simulink model "robot_arm_simul_utilization"  (R2017a)
settings: Solver=ode4  StartTime=0.0  StopTime=simul_time  FixedStep=delta  RelTol=1e-3
values from neighbouring files (symbols this model uses):
  B = 0    [Plot_utilization.m]
undefined symbols (not defined in the file or in its folder): A, A_, B_, C, C_, D, D_, delta, Dis_instant_P1, Dis_instant_P2, Dis_interval_P1, Dis_interval_P2, Dis_size_P1, Dis_size_P2, K, K_, L, L_, ref_P1, ref_P2
settings Model: Creator=sihoon  LastModifiedBy=root

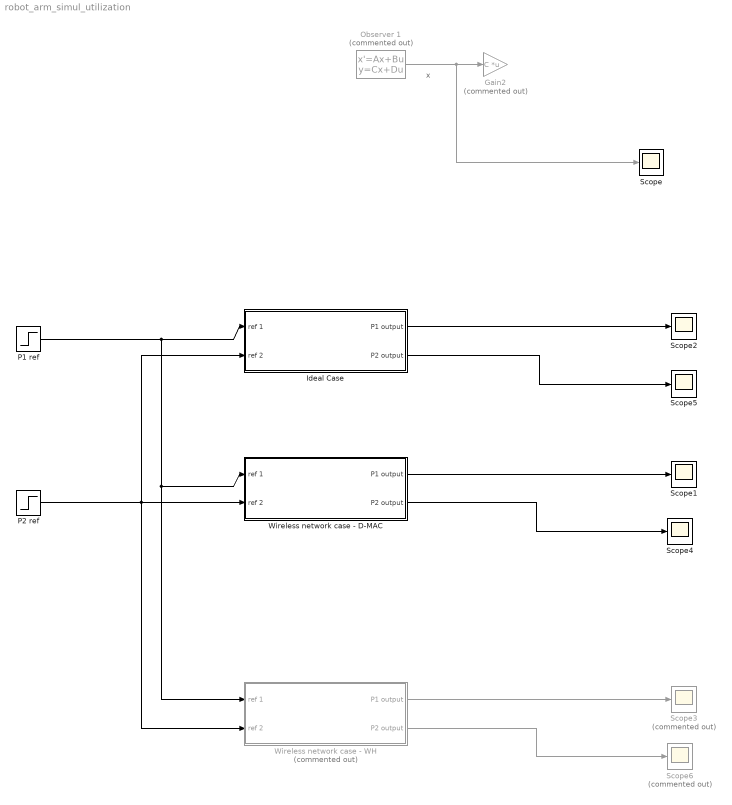
== system robot_arm_simul_utilization ==
  note: x
  Gain2 : Gain  Commented=on  Gain=C  Multiplication=Matrix(K*u)
  Ideal Case : Subsystem
  Observer 1 : StateSpace  Commented=on  A=A  B=B  C=eye(2)  D=[0; 0]  X0=0
  P1 ref : Step  Time=0  After=ref_P1  SampleTime=0
  P2 ref : Step  Time=0  After=ref_P2  SampleTime=0
  Scope{,1..2,4..5} (5 alike) : Scope
  Scope3 : Scope  Commented=on
  Scope6 : Scope  Commented=on
  Wireless network case - D-MAC : Subsystem
  "Wireless network case - WH " : Subsystem  Commented=on
  wires:
  Observer 1/1 -> Scope/1, Gain2/1
  Ideal Case/1(P1 output) -> Scope2/1
  Wireless network case - D-MAC/1(P1 output) -> Scope1/1
  P1 ref/1 -> "Wireless network case - WH "/1(ref 1), Wireless network case - D-MAC/1(ref 1), Ideal Case/1(ref 1)
  Wireless network case - D-MAC/2(P2 output) -> Scope4/1
  P2 ref/1 -> "Wireless network case - WH "/2(ref 2), Ideal Case/2(ref 2), Wireless network case - D-MAC/2(ref 2)
  Ideal Case/2(P2 output) -> Scope5/1
  "Wireless network case - WH "/1(P1 output) -> Scope3/1
  "Wireless network case - WH "/2(P2 output) -> Scope6/1

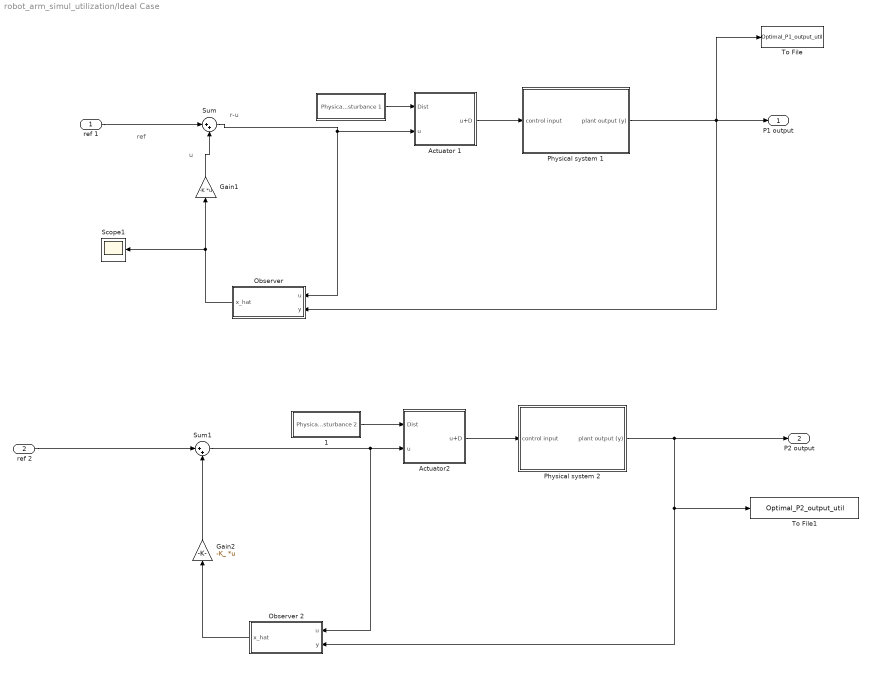
== system robot_arm_simul_utilization/Ideal Case ==
  note: u
  note: ref
  note: r-u
  ref 1 : Inport
  ref 2 : Inport  Port=2
  " " : Subsystem
  " 1" : Subsystem
  Actuator 1 : Subsystem
  Actuator2 : Subsystem
  Gain1 : Gain  Gain=-K  Multiplication=Matrix(K*u)
  Gain2 : Gain  Gain=-K_  Multiplication=Matrix(K*u)
  Observer : Subsystem
  Observer 2 : Subsystem
  Physical system 1 : Subsystem
  Physical system 2 : Subsystem
  Scope1 : Scope
  Sum : Sum  Inputs=|++
  Sum1 : Sum  Inputs=|++
  To File : ToFile  Filename=Optimal_P1_output_util  SaveFormat=Timeseries
  To File1 : ToFile  Filename=Optimal_P2_output_util  SaveFormat=Timeseries
  P1 output : Outport
  P2 output : Outport  Port=2
  wires:
  Physical system 1/1(plant output (y)) -> Observer/2(y), To File/1, P1 output/1
  Observer/1(x_hat) -> Scope1/1, Gain1/1
  ref 1/1 -> Sum/1
  Gain1/1 -> Sum/2
  Sum/1 -> Actuator 1/2(u), Observer/1(u)
  Actuator 1/1(u+D) -> Physical system 1/1(control input)
  " "/1(Physical Disturbance 1) -> Actuator 1/1(Dist)
  Actuator2/1(u+D) -> Physical system 2/1(control input)
  " 1"/1(Physical Disturbance 2) -> Actuator2/1(Dist)
  Physical system 2/1(plant output (y)) -> Observer 2/2(y), To File1/1, P2 output/1
  ref 2/1 -> Sum1/1
  Gain2/1 -> Sum1/2
  Observer 2/1(x_hat) -> Gain2/1
  Sum1/1 -> Observer 2/1(u), Actuator2/2(u)

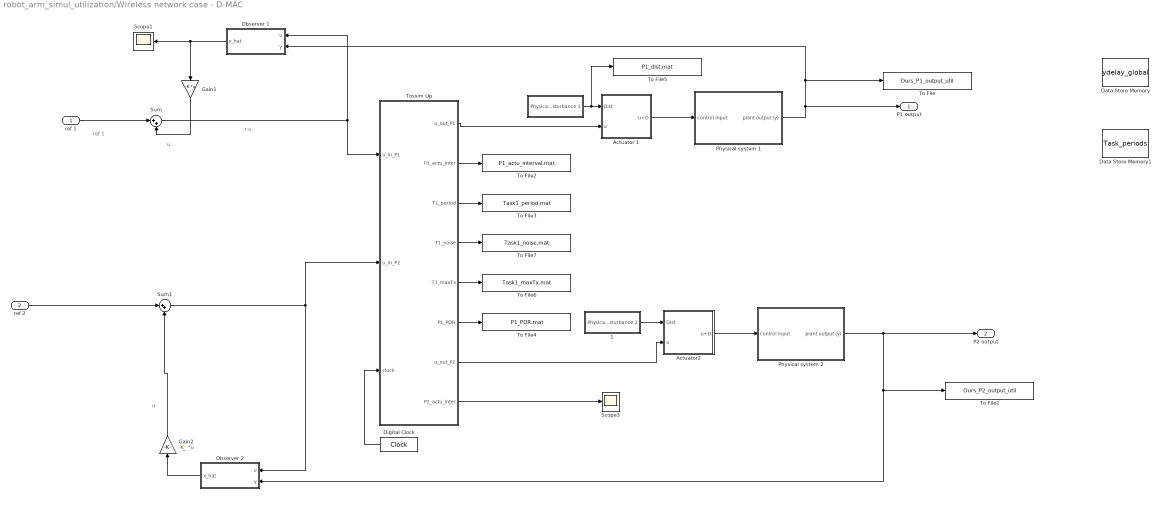
== system robot_arm_simul_utilization/Wireless network case - D-MAC ==
  note: u
  note: ref 1
  note: r-u
  note: u
  ref 1 : Inport
  ref 2 : Inport  Port=2
  " " : Subsystem
  " 1" : Subsystem
  Actuator 1 : Subsystem
  Actuator2 : Subsystem
  Data Store Memory : DataStoreMemory  DataStoreName=ydelay_global  ReadBeforeWriteMsg=warning  WriteAfterWriteMsg=warning  WriteAfterReadMsg=warning  InitialValue=[1; 1; 1; 1; 1; 1; 1; 1; 1; 1; 1; 1; 1; 1; 1]  ShowAdditionalParam=off  OutDataTypeStr=uint32
  Data Store Memory1 : DataStoreMemory  DataStoreName=Task_periods  ReadBeforeWriteMsg=warning  WriteAfterWriteMsg=warning  WriteAfterReadMsg=warning  InitialValue=Task_periods  ShowAdditionalParam=off  OutDataTypeStr=double
  Digital Clock : DigitalClock  SampleTime=delta
  Gain1 : Gain  Gain=-K  Multiplication=Matrix(K*u)
  Gain2 : Gain  Gain=-K_  Multiplication=Matrix(K*u)
  Observer 1 : Subsystem
  Observer 2 : Subsystem
  Physical system 1 : Subsystem
  Physical system 2 : Subsystem
  Scope1 : Scope
  Scope3 : Scope
  Sum : Sum  Inputs=|++
  Sum1 : Sum  Inputs=|++
  To File : ToFile  Filename=Ours_P1_output_util  SaveFormat=Timeseries
  To File1 : ToFile  Filename=Ours_P2_output_util  SaveFormat=Timeseries
  To File2 : ToFile  Filename=P1_actu_interval.mat  SaveFormat=Timeseries
  To File3 : ToFile  Filename=Task1_period.mat  SaveFormat=Timeseries
  To File4 : ToFile  Filename=P1_PDR.mat  SaveFormat=Timeseries
  To File5 : ToFile  Filename=P1_dist.mat  SaveFormat=Timeseries
  To File6 : ToFile  Filename=Task1_maxTx.mat  SaveFormat=Timeseries
  To File7 : ToFile  Filename=Task1_noise.mat  SaveFormat=Timeseries
  Tossim Up : MATLAB Function  TreatAsAtomicUnit=on
  P1 output : Outport
  P2 output : Outport  Port=2
  wires:
  ref 1/1 -> Sum/1
  Sum/1 -> Observer 1/1(u), Tossim Up/1(u_in_P1)
  Physical system 1/1(plant output (y)) -> Observer 1/2(y), To File/1, P1 output/1
  Gain1/1 -> Sum/2
  Observer 1/1(x_hat) -> Scope1/1, Gain1/1
  Tossim Up/7(u_out_P2) -> Actuator2/2(u)
  Digital Clock/1 -> Tossim Up/3(clock)
  Tossim Up/1(u_out_P1) -> Actuator 1/2(u)
  Actuator 1/1(u+D) -> Physical system 1/1(control input)
  " "/1(Physical Disturbance 1) -> To File5/1, Actuator 1/1(Dist)
  " 1"/1(Physical Disturbance 2) -> Actuator2/1(Dist)
  ref 2/1 -> Sum1/1
  Gain2/1 -> Sum1/2
  Observer 2/1(x_hat) -> Gain2/1
  Actuator2/1(u+D) -> Physical system 2/1(control input)
  Physical system 2/1(plant output (y)) -> To File1/1, Observer 2/2(y), P2 output/1
  Sum1/1 -> Observer 2/1(u), Tossim Up/2(u_in_P2)
  Tossim Up/2(P1_actu_inter) -> To File2/1
  Tossim Up/8(P2_actu_inter) -> Scope3/1
  Tossim Up/3(T1_period) -> To File3/1
  Tossim Up/6(P1_PDR) -> To File4/1
  Tossim Up/5(T1_maxTx) -> To File6/1
  Tossim Up/4(T1_noise) -> To File7/1

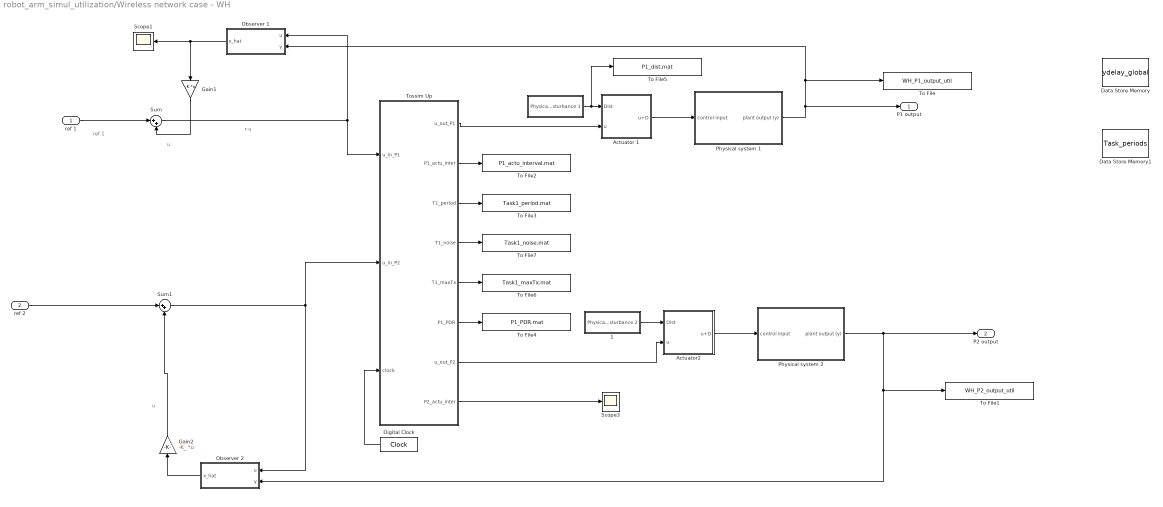
== system robot_arm_simul_utilization/Wireless network case - WH  ==
  note: u
  note: ref 1
  note: r-u
  note: u
  ref 1 : Inport
  ref 2 : Inport  Port=2
  " " : Subsystem
  " 1" : Subsystem
  Actuator 1 : Subsystem
  Actuator2 : Subsystem
  Data Store Memory : DataStoreMemory  DataStoreName=ydelay_global  ReadBeforeWriteMsg=warning  WriteAfterWriteMsg=warning  WriteAfterReadMsg=warning  InitialValue=[1; 1; 1; 1; 1; 1; 1; 1; 1; 1; 1; 1; 1; 1; 1]  ShowAdditionalParam=off  OutDataTypeStr=uint32
  Data Store Memory1 : DataStoreMemory  DataStoreName=Task_periods  ReadBeforeWriteMsg=warning  WriteAfterWriteMsg=warning  WriteAfterReadMsg=warning  InitialValue=Task_periods  ShowAdditionalParam=off  OutDataTypeStr=double
  Digital Clock : DigitalClock  SampleTime=delta
  Gain1 : Gain  Gain=-K  Multiplication=Matrix(K*u)
  Gain2 : Gain  Gain=-K_  Multiplication=Matrix(K*u)
  Observer 1 : Subsystem
  Observer 2 : Subsystem
  Physical system 1 : Subsystem
  Physical system 2 : Subsystem
  Scope1 : Scope
  Scope3 : Scope
  Sum : Sum  Inputs=|++
  Sum1 : Sum  Inputs=|++
  To File : ToFile  Filename=WH_P1_output_util  SaveFormat=Timeseries
  To File1 : ToFile  Filename=WH_P2_output_util  SaveFormat=Timeseries
  To File2 : ToFile  Filename=P1_actu_interval.mat  SaveFormat=Timeseries
  To File3 : ToFile  Filename=Task1_period.mat  SaveFormat=Timeseries
  To File4 : ToFile  Filename=P1_PDR.mat  SaveFormat=Timeseries
  To File5 : ToFile  Filename=P1_dist.mat  SaveFormat=Timeseries
  To File6 : ToFile  Filename=Task1_maxTx.mat  SaveFormat=Timeseries
  To File7 : ToFile  Filename=Task1_noise.mat  SaveFormat=Timeseries
  Tossim Up : MATLAB Function  TreatAsAtomicUnit=on
  P1 output : Outport
  P2 output : Outport  Port=2
  wires:
  ref 1/1 -> Sum/1
  Sum/1 -> Observer 1/1(u), Tossim Up/1(u_in_P1)
  Physical system 1/1(plant output (y)) -> Observer 1/2(y), To File/1, P1 output/1
  Gain1/1 -> Sum/2
  Observer 1/1(x_hat) -> Scope1/1, Gain1/1
  Tossim Up/7(u_out_P2) -> Actuator2/2(u)
  Digital Clock/1 -> Tossim Up/3(clock)
  Tossim Up/1(u_out_P1) -> Actuator 1/2(u)
  Actuator 1/1(u+D) -> Physical system 1/1(control input)
  " "/1(Physical Disturbance 1) -> To File5/1, Actuator 1/1(Dist)
  " 1"/1(Physical Disturbance 2) -> Actuator2/1(Dist)
  ref 2/1 -> Sum1/1
  Gain2/1 -> Sum1/2
  Observer 2/1(x_hat) -> Gain2/1
  Actuator2/1(u+D) -> Physical system 2/1(control input)
  Physical system 2/1(plant output (y)) -> To File1/1, Observer 2/2(y), P2 output/1
  Sum1/1 -> Observer 2/1(u), Tossim Up/2(u_in_P2)
  Tossim Up/2(P1_actu_inter) -> To File2/1
  Tossim Up/8(P2_actu_inter) -> Scope3/1
  Tossim Up/3(T1_period) -> To File3/1
  Tossim Up/6(P1_PDR) -> To File4/1
  Tossim Up/5(T1_maxTx) -> To File6/1
  Tossim Up/4(T1_noise) -> To File7/1

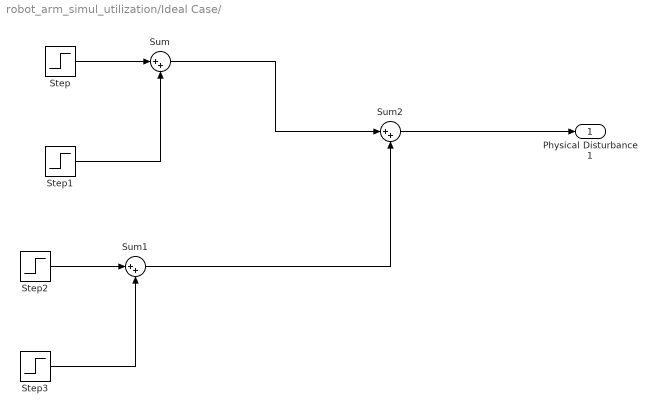
== system robot_arm_simul_utilization/Ideal Case/  ==
  Step : Step  Time=Dis_instant_P1  After=Dis_size_P1  SampleTime=0
  Step1 : Step  Time=Dis_instant_P1+(Dis_interval_P1*1/2)  After=-Dis_size_P1  SampleTime=0
  Step2 : Step  Time=Dis_instant_P1+(Dis_interval_P1*1/2)  After=-Dis_size_P1  SampleTime=0
  Step3 : Step  Time=Dis_instant_P1+Dis_interval_P1  After=Dis_size_P1  SampleTime=0
  Sum : Sum  Inputs=|++
  Sum1 : Sum  Inputs=|++
  Sum2 : Sum  Inputs=|++
  Physical Disturbance 1 : Outport
  wires:
  Step/1 -> Sum/1
  Step1/1 -> Sum/2
  Sum1/1 -> Sum2/2
  Step2/1 -> Sum1/1
  Step3/1 -> Sum1/2
  Sum/1 -> Sum2/1
  Sum2/1 -> Physical Disturbance 1/1

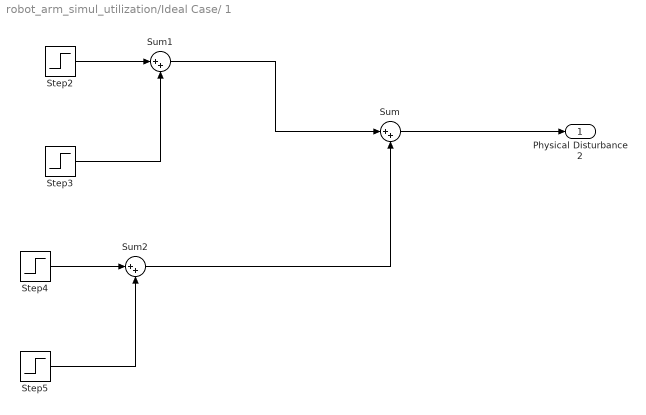
== system robot_arm_simul_utilization/Ideal Case/ 1 ==
  Step2 : Step  Time=Dis_instant_P2  After=Dis_size_P2  SampleTime=0
  Step3 : Step  Time=Dis_instant_P2+(Dis_interval_P2*1/2)  After=-Dis_size_P2  SampleTime=0
  Step4 : Step  Time=Dis_instant_P2+(Dis_interval_P2*1/2)  After=-Dis_size_P2  SampleTime=0
  Step5 : Step  Time=Dis_instant_P2+Dis_interval_P2  After=Dis_size_P2  SampleTime=0
  Sum : Sum  Inputs=|++
  Sum1 : Sum  Inputs=|++
  Sum2 : Sum  Inputs=|++
  Physical Disturbance 2 : Outport
  wires:
  Sum/1 -> Physical Disturbance 2/1
  Step2/1 -> Sum1/1
  Sum2/1 -> Sum/2
  Step4/1 -> Sum2/1
  Step5/1 -> Sum2/2
  Sum1/1 -> Sum/1
  Step3/1 -> Sum1/2

== system robot_arm_simul_utilization/Ideal Case/Actuator 1 ==
  Dist : Inport
  u : Inport  Port=2
  Sum : Sum  Inputs=|++
  u+D : Outport
  wires:
  u/1 -> Sum/2
  Dist/1 -> Sum/1
  Sum/1 -> u+D/1

== system robot_arm_simul_utilization/Ideal Case/Actuator2 ==
  Dist : Inport
  u : Inport  Port=2
  Sum : Sum  Inputs=|++
  u+D : Outport
  wires:
  u/1 -> Sum/2
  Dist/1 -> Sum/1
  Sum/1 -> u+D/1

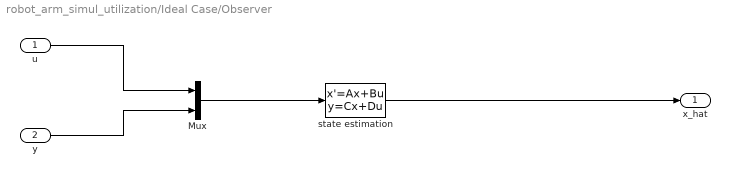
== system robot_arm_simul_utilization/Ideal Case/Observer ==
  u : Inport
  y : Inport  Port=2
  Mux : Mux  Inputs=2
  "state estimation " : StateSpace  A=A-L*C  B=[B L]  C=eye(2)  D=[0 0;0 0]  X0=0
  x_hat : Outport
  wires:
  u/1 -> Mux/1
  y/1 -> Mux/2
  Mux/1 -> "state estimation "/1
  "state estimation "/1 -> x_hat/1

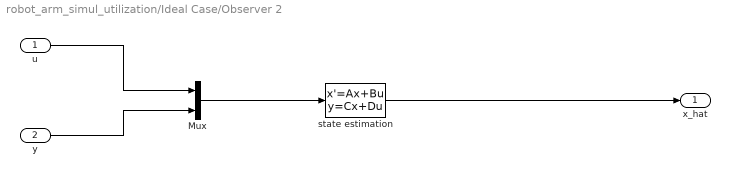
== system robot_arm_simul_utilization/Ideal Case/Observer 2 ==
  u : Inport
  y : Inport  Port=2
  Mux : Mux  Inputs=2
  "state estimation " : StateSpace  A=A_-L_*C_  B=[B_ L_]  C=eye(2)  D=[0 0;0 0]  X0=0
  x_hat : Outport
  wires:
  u/1 -> Mux/1
  y/1 -> Mux/2
  Mux/1 -> "state estimation "/1
  "state estimation "/1 -> x_hat/1

== system robot_arm_simul_utilization/Ideal Case/Physical system 1 ==
  control input : Inport
  robot_arm system : S-Function  FunctionName=robot_arm_dynamics  Parameters=A,B,C,D  SFunctionDeploymentMode=off  EnableBusSupport=off
  plant output (y) : Outport
  wires:
  control input/1 -> robot_arm system/1
  robot_arm system/1 -> plant output (y)/1

== system robot_arm_simul_utilization/Ideal Case/Physical system 2 ==
  control input : Inport
  robot_arm system : S-Function  FunctionName=robot_arm_dynamics2  Parameters=A_,B_,C_,D_  SFunctionDeploymentMode=off  EnableBusSupport=off
  plant output (y) : Outport
  wires:
  control input/1 -> robot_arm system/1
  robot_arm system/1 -> plant output (y)/1

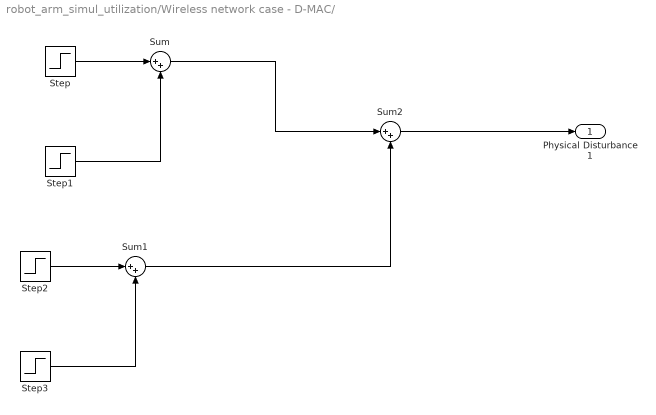
== system robot_arm_simul_utilization/Wireless network case - D-MAC/  ==
  Step : Step  Time=Dis_instant_P1  After=Dis_size_P1  SampleTime=0
  Step1 : Step  Time=Dis_instant_P1+(Dis_interval_P1*1/2)  After=-Dis_size_P1  SampleTime=0
  Step2 : Step  Time=Dis_instant_P1+(Dis_interval_P1*1/2)  After=-Dis_size_P1  SampleTime=0
  Step3 : Step  Time=Dis_instant_P1+Dis_interval_P1  After=Dis_size_P1  SampleTime=0
  Sum : Sum  Inputs=|++
  Sum1 : Sum  Inputs=|++
  Sum2 : Sum  Inputs=|++
  Physical Disturbance 1 : Outport
  wires:
  Step/1 -> Sum/1
  Step1/1 -> Sum/2
  Sum1/1 -> Sum2/2
  Step2/1 -> Sum1/1
  Step3/1 -> Sum1/2
  Sum/1 -> Sum2/1
  Sum2/1 -> Physical Disturbance 1/1

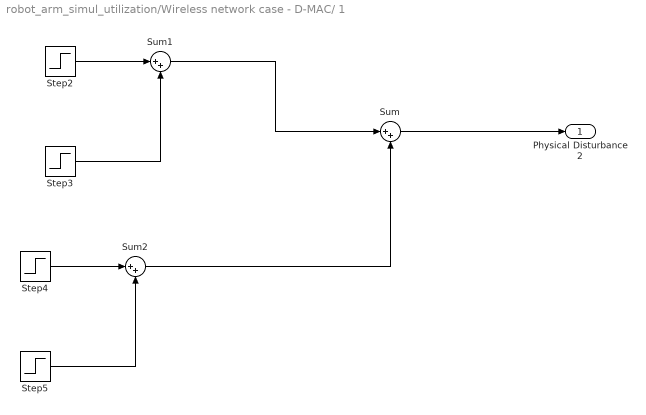
== system robot_arm_simul_utilization/Wireless network case - D-MAC/ 1 ==
  Step2 : Step  Time=Dis_instant_P2  After=Dis_size_P2  SampleTime=0
  Step3 : Step  Time=Dis_instant_P2+(Dis_interval_P2*1/2)  After=-Dis_size_P2  SampleTime=0
  Step4 : Step  Time=Dis_instant_P2+(Dis_interval_P2*1/2)  After=-Dis_size_P2  SampleTime=0
  Step5 : Step  Time=Dis_instant_P2+Dis_interval_P2  After=Dis_size_P2  SampleTime=0
  Sum : Sum  Inputs=|++
  Sum1 : Sum  Inputs=|++
  Sum2 : Sum  Inputs=|++
  Physical Disturbance 2 : Outport
  wires:
  Sum/1 -> Physical Disturbance 2/1
  Step2/1 -> Sum1/1
  Sum2/1 -> Sum/2
  Step4/1 -> Sum2/1
  Step5/1 -> Sum2/2
  Sum1/1 -> Sum/1
  Step3/1 -> Sum1/2

== system robot_arm_simul_utilization/Wireless network case - D-MAC/Actuator 1 ==
  Dist : Inport
  u : Inport  Port=2
  Sum : Sum  Inputs=|++
  u+D : Outport
  wires:
  u/1 -> Sum/2
  Dist/1 -> Sum/1
  Sum/1 -> u+D/1

== system robot_arm_simul_utilization/Wireless network case - D-MAC/Actuator2 ==
  Dist : Inport
  u : Inport  Port=2
  Sum : Sum  Inputs=|++
  u+D : Outport
  wires:
  u/1 -> Sum/2
  Dist/1 -> Sum/1
  Sum/1 -> u+D/1

== system robot_arm_simul_utilization/Wireless network case - D-MAC/Observer 1 ==
  u : Inport
  y : Inport  Port=2
  Mux : Mux  Inputs=2
  "state estimation " : StateSpace  A=A-L*C  B=[B L]  C=eye(2)  D=[0 0;0 0]  X0=0
  x_hat : Outport
  wires:
  u/1 -> Mux/1
  y/1 -> Mux/2
  Mux/1 -> "state estimation "/1
  "state estimation "/1 -> x_hat/1

== system robot_arm_simul_utilization/Wireless network case - D-MAC/Observer 2 ==
  u : Inport
  y : Inport  Port=2
  Mux : Mux  Inputs=2
  "state estimation " : StateSpace  A=A_-L_*C_  B=[B_ L_]  C=eye(2)  D=[0 0;0 0]  X0=0
  x_hat : Outport
  wires:
  u/1 -> Mux/1
  y/1 -> Mux/2
  Mux/1 -> "state estimation "/1
  "state estimation "/1 -> x_hat/1

== system robot_arm_simul_utilization/Wireless network case - D-MAC/Physical system 1 ==
  control input : Inport
  robot_arm system : S-Function  FunctionName=robot_arm_dynamics  Parameters=A,B,C,D  SFunctionDeploymentMode=off  EnableBusSupport=off
  plant output (y) : Outport
  wires:
  control input/1 -> robot_arm system/1
  robot_arm system/1 -> plant output (y)/1

== system robot_arm_simul_utilization/Wireless network case - D-MAC/Physical system 2 ==
  control input : Inport
  robot_arm system : S-Function  FunctionName=robot_arm_dynamics2  Parameters=A_,B_,C_,D_  SFunctionDeploymentMode=off  EnableBusSupport=off
  plant output (y) : Outport
  wires:
  control input/1 -> robot_arm system/1
  robot_arm system/1 -> plant output (y)/1

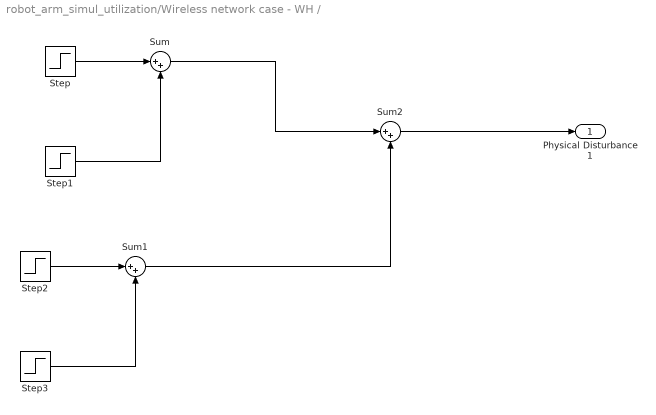
== system robot_arm_simul_utilization/Wireless network case - WH /  ==
  Step : Step  Time=Dis_instant_P1  After=Dis_size_P1  SampleTime=0
  Step1 : Step  Time=Dis_instant_P1+(Dis_interval_P1*1/2)  After=-Dis_size_P1  SampleTime=0
  Step2 : Step  Time=Dis_instant_P1+(Dis_interval_P1*1/2)  After=-Dis_size_P1  SampleTime=0
  Step3 : Step  Time=Dis_instant_P1+Dis_interval_P1  After=Dis_size_P1  SampleTime=0
  Sum : Sum  Inputs=|++
  Sum1 : Sum  Inputs=|++
  Sum2 : Sum  Inputs=|++
  Physical Disturbance 1 : Outport
  wires:
  Step/1 -> Sum/1
  Step1/1 -> Sum/2
  Sum1/1 -> Sum2/2
  Step2/1 -> Sum1/1
  Step3/1 -> Sum1/2
  Sum/1 -> Sum2/1
  Sum2/1 -> Physical Disturbance 1/1

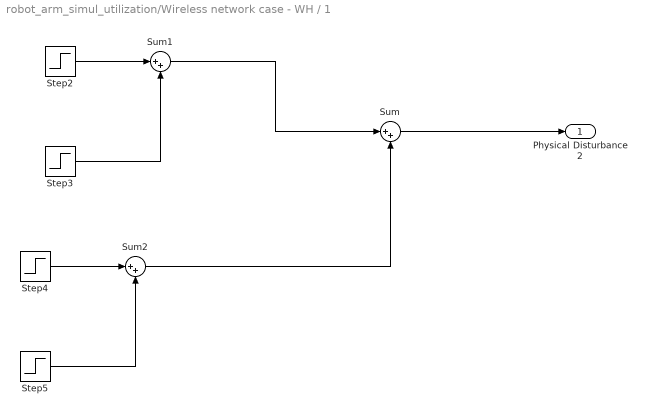
== system robot_arm_simul_utilization/Wireless network case - WH / 1 ==
  Step2 : Step  Time=Dis_instant_P2  After=Dis_size_P2  SampleTime=0
  Step3 : Step  Time=Dis_instant_P2+(Dis_interval_P2*1/2)  After=-Dis_size_P2  SampleTime=0
  Step4 : Step  Time=Dis_instant_P2+(Dis_interval_P2*1/2)  After=-Dis_size_P2  SampleTime=0
  Step5 : Step  Time=Dis_instant_P2+Dis_interval_P2  After=Dis_size_P2  SampleTime=0
  Sum : Sum  Inputs=|++
  Sum1 : Sum  Inputs=|++
  Sum2 : Sum  Inputs=|++
  Physical Disturbance 2 : Outport
  wires:
  Sum/1 -> Physical Disturbance 2/1
  Step2/1 -> Sum1/1
  Sum2/1 -> Sum/2
  Step4/1 -> Sum2/1
  Step5/1 -> Sum2/2
  Sum1/1 -> Sum/1
  Step3/1 -> Sum1/2

== system robot_arm_simul_utilization/Wireless network case - WH /Actuator 1 ==
  Dist : Inport
  u : Inport  Port=2
  Sum : Sum  Inputs=|++
  u+D : Outport
  wires:
  u/1 -> Sum/2
  Dist/1 -> Sum/1
  Sum/1 -> u+D/1

== system robot_arm_simul_utilization/Wireless network case - WH /Actuator2 ==
  Dist : Inport
  u : Inport  Port=2
  Sum : Sum  Inputs=|++
  u+D : Outport
  wires:
  u/1 -> Sum/2
  Dist/1 -> Sum/1
  Sum/1 -> u+D/1

== system robot_arm_simul_utilization/Wireless network case - WH /Observer 1 ==
  u : Inport
  y : Inport  Port=2
  Mux : Mux  Inputs=2
  "state estimation " : StateSpace  A=A-L*C  B=[B L]  C=eye(2)  D=[0 0;0 0]  X0=0
  x_hat : Outport
  wires:
  u/1 -> Mux/1
  y/1 -> Mux/2
  Mux/1 -> "state estimation "/1
  "state estimation "/1 -> x_hat/1

== system robot_arm_simul_utilization/Wireless network case - WH /Observer 2 ==
  u : Inport
  y : Inport  Port=2
  Mux : Mux  Inputs=2
  "state estimation " : StateSpace  A=A_-L_*C_  B=[B_ L_]  C=eye(2)  D=[0 0;0 0]  X0=0
  x_hat : Outport
  wires:
  u/1 -> Mux/1
  y/1 -> Mux/2
  Mux/1 -> "state estimation "/1
  "state estimation "/1 -> x_hat/1

== system robot_arm_simul_utilization/Wireless network case - WH /Physical system 1 ==
  control input : Inport
  robot_arm system : S-Function  FunctionName=robot_arm_dynamics  Parameters=A,B,C,D  SFunctionDeploymentMode=off  EnableBusSupport=off
  plant output (y) : Outport
  wires:
  control input/1 -> robot_arm system/1
  robot_arm system/1 -> plant output (y)/1

== system robot_arm_simul_utilization/Wireless network case - WH /Physical system 2 ==
  control input : Inport
  robot_arm system : S-Function  FunctionName=robot_arm_dynamics2  Parameters=A_,B_,C_,D_  SFunctionDeploymentMode=off  EnableBusSupport=off
  plant output (y) : Outport
  wires:
  control input/1 -> robot_arm system/1
  robot_arm system/1 -> plant output (y)/1

== matlab function robot_arm_simul_utilization/Wireless network case - D-MAC/Tossim Up ==
  settings: updateMethod=DISCRETE
  data: u_out_P1 output; P1_actu_inter output; T1_period output; T1_noise output; T1_maxTx output; P1_PDR output; u_out_P2 output; u_in_P1 input; ydelay_global data_store_memory; u_in_P2 input; clock input; P2_actu_inter output; Task_periods data_store_memory
function [u_out_P1, P1_actu_inter, T1_period, T1_noise, T1_maxTx, P1_PDR, u_out_P2, P2_actu_inter]  = Tossim_block(u_in_P1, u_in_P2, clock)
% Inputs:
% ymea: measurement from structure
% Outputs:
% ymea1: measurement output
% ydelay: delay traces
persistent tmp_u_in_P1 tmp_u_in_P2 prev_u_out_P1 prev_u_out_P2    % delay trace
persistent prev_P1_actu_inter prev_P2_actu_inter prev_P1_clock prev_P2_clock % inter arrival time
persistent tmp_T1_period tmp_T2_period tmp_rcv_flag1 period_cunt1 windowbuff windowsize
persistent tmp_T1_maxTx tmp_T1_noise
persistent i                 % count 
persistent tossim_flag
global ydelay_global delta Task_periods


% allow these matlab functions to be used in Embedded Matlab block
eml.extrinsic('python');
eml.extrinsic('num2str');
eml.extrinsic('str2num');
eml.extrinsic('delay_summary');
eml.extrinsic('disp');
eml.extrinsic('ps_aggregation');
eml.extrinsic('for');
eml.extrinsic('end');

if isempty(i)
    i = 0;
    %past_ymea = 0;
    tmp_u_in_P1 = u_in_P1;
    tmp_u_in_P2 = u_in_P2;
    prev_u_out_P1 = 0;
    prev_u_out_P2 = 0;
    tossim_flag = 0;
    prev_P1_actu_inter = 0;
    prev_P2_actu_inter = 0;
    prev_P1_clock = 0;
    prev_P2_clock = 0;
    P1_actu_inter = 0;
    P2_actu_inter = 0;
    tmp_T1_period = 0;
    tmp_T2_period = 0;
    tmp_rcv_flag1 = 0;
    period_cunt1 = 0;
    windowsize = 20;
    windowbuff = zeros(1,windowsize);
    tmp_T1_maxTx = 0;
    tmp_T1_noise = 0;
end
i = i+1;

%[row column] = size(Task_period_time);

ydelay = [1 0 0 0 0 0 0 0 0]';
% call python to communicate with TOSSIM

% where clock increase with 1ms period
TOSSIM_step_size = 0.01;  % 10ms

call_count = 1; %Superframelength
rssi = -69;%sensor rssi

%% Tossim results 
% run Tossim once every 10ms
if mod(clock, TOSSIM_step_size) == 0
    if tossim_flag == 0
        tossim_flag = tossim_flag + 1;
        clock;
        [resultz] = ps_aggregation(call_count, rssi, clock); %here call TOSSIM Client ----yh
        end_to_end_delivery_result_aggregated = sum(resultz);
        [delay] = delay_summary(resultz);
        ydelay = delay';
        resultz;
        
        % Check T1 Period %
        tmp_T1_period = resultz(1,8) / 100; % convert into ms
        % Check T1 maxTx %
        tmp_T1_maxTx = resultz(1,7);
        % Check noise %
        tmp_T1_noise = resultz(1,6);
        
        %% Check P1 actuation PDR
        % Check T1 receive in a period %   
        if ydelay(2,1) == 1     % Task1 receive
            tmp_rcv_flag1 = 1;
        end
        
        % for calculating PDR and for updating u_in_P1
        if mod(clock, tmp_T1_period) == 0 
            % PDR 
            tmp_period_cunt1 = mod(period_cunt1, windowsize);
            if tmp_rcv_flag1 == 1
                windowbuff(1,tmp_period_cunt1+1) = 1;
            else
                windowbuff(1,tmp_period_cunt1+1) = 0;
            end
            period_cunt1 = period_cunt1 + 1;
            tmp_rcv_flag1 = 0;
            
            % update
            tmp_u_in_P1 = u_in_P1;
        end
        
        % P2 u update
        tmp_T2_period = Task_periods(2,1)*0.01;
        if mod(clock, tmp_T2_period) == 0
            tmp_u_in_P2 = u_in_P2;
        end

        
    else
        resultz = [0 0 0 0 0 0 0 0];
        [delay] = delay_summary(resultz);
        ydelay = delay';
    end
else
    tossim_flag = 0;
    resultz = [0 0 0 0 0 0 0 0];
    [delay] = delay_summary(resultz);
    ydelay = delay';
end



%% Outputs
for i_yg = 1:9
    ydelay_global(i_yg, 1) = ydelay(i_yg, 1);
end
delay = ydelay';

task1_index = 1;
task2_index = 2;
if delay(1,task1_index + 1)~=88
    u_out_P1 = tmp_u_in_P1;
    prev_u_out_P1 = u_out_P1;
    u_out_P2 = prev_u_out_P2;
    %%%%
    P1_actu_inter = clock - prev_P1_clock;
    prev_P1_clock = clock;
    prev_P1_actu_inter = P1_actu_inter;
    P2_actu_inter = prev_P2_actu_inter;
elseif delay(1,task2_index + 1)~=88
    u_out_P2 = tmp_u_in_P2;
    prev_u_out_P2 = u_out_P2;
    u_out_P1 = prev_u_out_P1;
    %%%
    P2_actu_inter = clock - prev_P2_clock;
    prev_P2_clock = clock;
    prev_P2_actu_inter = P2_actu_inter;
    P1_actu_inter = prev_P1_actu_inter;
else
    u_out_P1 = prev_u_out_P1;
    u_out_P2 = prev_u_out_P2;
    P1_actu_inter = prev_P1_actu_inter;
    P2_actu_inter = prev_P2_actu_inter;
end

T1_period = tmp_T1_period;
P1_PDR = sum(windowbuff)/windowsize;
T1_maxTx = tmp_T1_maxTx;
T1_noise = tmp_T1_noise;
end

== matlab function robot_arm_simul_utilization/Wireless network case - WH /Tossim Up ==
  settings: updateMethod=DISCRETE
  data: u_out_P1 output; P1_actu_inter output; T1_period output; T1_noise output; T1_maxTx output; P1_PDR output; u_out_P2 output; u_in_P1 input; ydelay_global data_store_memory; u_in_P2 input; clock input; P2_actu_inter output; Task_periods data_store_memory
function [u_out_P1, P1_actu_inter, T1_period, T1_noise, T1_maxTx, P1_PDR, u_out_P2, P2_actu_inter]  = Tossim_block(u_in_P1, u_in_P2, clock)
% Inputs:
% ymea: measurement from structure
% Outputs:
% ymea1: measurement output
% ydelay: delay traces
persistent tmp_u_in_P1 tmp_u_in_P2 prev_u_out_P1 prev_u_out_P2    % delay trace
persistent prev_P1_actu_inter prev_P2_actu_inter prev_P1_clock prev_P2_clock % inter arrival time
persistent tmp_T1_period tmp_T2_period tmp_rcv_flag1 period_cunt1 windowbuff windowsize
persistent tmp_T1_maxTx tmp_T1_noise
persistent i                 % count 
persistent tossim_flag
global ydelay_global delta Task_periods


% allow these matlab functions to be used in Embedded Matlab block
eml.extrinsic('python');
eml.extrinsic('num2str');
eml.extrinsic('str2num');
eml.extrinsic('delay_summary');
eml.extrinsic('disp');
eml.extrinsic('ps_aggregation');
eml.extrinsic('for');
eml.extrinsic('end');

if isempty(i)
    i = 0;
    %past_ymea = 0;
    tmp_u_in_P1 = u_in_P1;
    tmp_u_in_P2 = u_in_P2;
    prev_u_out_P1 = 0;
    prev_u_out_P2 = 0;
    tossim_flag = 0;
    prev_P1_actu_inter = 0;
    prev_P2_actu_inter = 0;
    prev_P1_clock = 0;
    prev_P2_clock = 0;
    P1_actu_inter = 0;
    P2_actu_inter = 0;
    tmp_T1_period = 0;
    tmp_T2_period = 0;
    tmp_rcv_flag1 = 0;
    period_cunt1 = 0;
    windowsize = 20;
    windowbuff = zeros(1,windowsize);
    tmp_T1_maxTx = 0;
    tmp_T1_noise = 0;
end
i = i+1;

%[row column] = size(Task_period_time);

ydelay = [1 0 0 0 0 0 0 0 0]';
% call python to communicate with TOSSIM

% where clock increase with 1ms period
TOSSIM_step_size = 0.01;  % 10ms

call_count = 1; %Superframelength
rssi = -69;%sensor rssi

%% Tossim results 
% run Tossim once every 10ms
if mod(clock, TOSSIM_step_size) == 0
    if tossim_flag == 0
        tossim_flag = tossim_flag + 1;
        clock;
        [resultz] = ps_aggregation(call_count, rssi, clock); %here call TOSSIM Client ----yh
        end_to_end_delivery_result_aggregated = sum(resultz);
        [delay] = delay_summary(resultz);
        ydelay = delay';
        resultz;
        
        % Check T1 Period %
        %tmp_T1_period = resultz(1,8) / 100 % convert into ms
        % Check T1 maxTx %
        tmp_T1_maxTx = resultz(1,7);
        % Check noise %
        tmp_T1_noise = resultz(1,6);
        
        %% Check P1 actuation PDR
        % Check T1 receive in a period %   
        if ydelay(2,1) == 1     % Task1 receive
            tmp_rcv_flag1 = 1;
        end
        
        tmp_T1_period = Task_periods(1,1)*0.01;
        % for calculating PDR and for updating u_in_P1
        if mod(clock, tmp_T1_period) == 0 
            % PDR 
            tmp_period_cunt1 = mod(period_cunt1, windowsize);
            if tmp_rcv_flag1 == 1
                windowbuff(1,tmp_period_cunt1+1) = 1;
            else
                windowbuff(1,tmp_period_cunt1+1) = 0;
            end
            period_cunt1 = period_cunt1 + 1;
            tmp_rcv_flag1 = 0;
            
            % update
            tmp_u_in_P1 = u_in_P1;
        end
        
        % P2 u update
        tmp_T2_period = Task_periods(2,1)*0.01;
        if mod(clock, tmp_T2_period) == 0
            tmp_u_in_P2 = u_in_P2;
        end
        

        
    else
        resultz = [0 0 0 0 0 0 0 0];
        [delay] = delay_summary(resultz);
        ydelay = delay';
    end
else
    tossim_flag = 0;
    resultz = [0 0 0 0 0 0 0 0];
    [delay] = delay_summary(resultz);
    ydelay = delay';
end



%% Outputs
for i_yg = 1:9
    ydelay_global(i_yg, 1) = ydelay(i_yg, 1);
end
delay = ydelay';

task1_index = 1;
task2_index = 2;
if delay(1,task1_index + 1)~=88
    u_out_P1 = tmp_u_in_P1;
    prev_u_out_P1 = u_out_P1;
    u_out_P2 = prev_u_out_P2;
    %%%%
    P1_actu_inter = clock - prev_P1_clock;
    prev_P1_clock = clock;
    prev_P1_actu_inter = P1_actu_inter;
    P2_actu_inter = prev_P2_actu_inter;
elseif delay(1,task2_index + 1)~=88
    u_out_P2 = tmp_u_in_P2;
    prev_u_out_P2 = u_out_P2;
    u_out_P1 = prev_u_out_P1;
    %%%
    P2_actu_inter = clock - prev_P2_clock;
    prev_P2_clock = clock;
    prev_P2_actu_inter = P2_actu_inter;
    P1_actu_inter = prev_P1_actu_inter;
else
    u_out_P1 = prev_u_out_P1;
    u_out_P2 = prev_u_out_P2;
    P1_actu_inter = prev_P1_actu_inter;
    P2_actu_inter = prev_P2_actu_inter;
end

T1_period = tmp_T1_period;
P1_PDR = sum(windowbuff)/windowsize;
T1_maxTx = tmp_T1_maxTx;
T1_noise = tmp_T1_noise;
end
